simulink library "EngineModelsLibrary"  (R2014b)
settings: Solver=ode45  StartTime=0.0  StopTime=10.0  RelTol=1e-3
values from neighbouring files (symbols this model uses):
  k = 0.2    [ES_Run.m]    (also in ES_Run_v2.m = 10)
undefined symbols (not defined in the file or in its folder): b, COBRA_Compressor, cp, CPT_COBRA_LIB, D, etalim, gam, Newton, Pa, PARAM, Pl, pref, Ps, R, Raphson, rlim, T_0, Tref, Wclim
undefined symbols (not defined in the file): cr, e, etagain, fit_pars, kL, kS, par
(part 3 of 3)

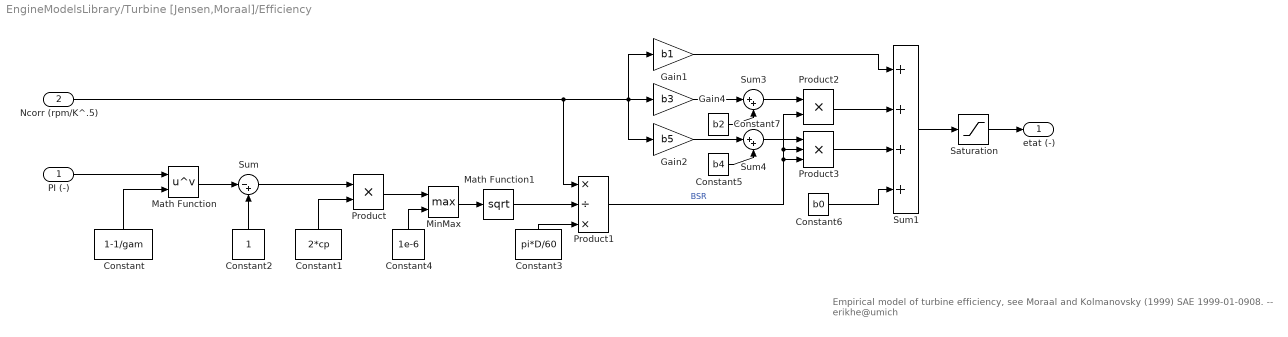
== system EngineModelsLibrary/Turbine [Jensen,Moraal]/Efficiency ==
  note: Empirical model of turbine efficiency, see Moraal and Kolmanovsky (1999) SAE 1999-01-0908.
      |  -- erikhe@umich
  PI (-) : Inport
  Ncorr (rpm/K^.5) : Inport  Port=2
  Constant : Constant  Value=1-1/gam
  Constant1 : Constant  Value=2*cp
  Constant2 : Constant
  Constant3 : Constant  Value=pi*D/60
  Constant4 : Constant  Value=1e-6
  Constant5 : Constant  Value=b4
  Constant6 : Constant  Value=b0
  Constant7 : Constant  Value=b2
  Gain1 : Gain  Gain=b1
  Gain2 : Gain  Gain=b5
  Gain4 : Gain  Gain=b3
  Math Function : Math  Operator=pow  SaturateOnIntegerOverflow=on
  Math Function1 : Math  Operator=sqrt  SaturateOnIntegerOverflow=on
  MinMax : MinMax  Function=max  Inputs=2
  Product : Product  RndMeth=Zero
  Product1 : Product  Inputs=*/*  RndMeth=Zero
  Product2 : Product  RndMeth=Zero
  Product3 : Product  Inputs=3  RndMeth=Zero
  Saturation : Saturate  UpperLimit=etamax  LowerLimit=etamin
  Sum : Sum  Inputs=|-+
  Sum1 : Sum  Inputs=4
  Sum3 : Sum  Inputs=|++
  Sum4 : Sum  Inputs=|++
  etat (-) : Outport
  wires:
  Product1/1 -> Product3/3, Product3/2, Product2/2  "BSR"
  Constant6/1 -> Sum1/4
  Product2/1 -> Sum1/2
  Product3/1 -> Sum1/3
  Sum4/1 -> Product3/1
  Sum3/1 -> Product2/1
  Gain1/1 -> Sum1/1
  Constant5/1 -> Sum4/2
  Constant7/1 -> Sum3/2
  Gain2/1 -> Sum4/1
  Gain4/1 -> Sum3/1
  Saturation/1 -> etat (-)/1
  Sum1/1 -> Saturation/1
  Ncorr (rpm/K^.5)/1 -> Gain1/1, Gain2/1, Gain4/1, Product1/1
  Constant3/1 -> Product1/3
  Constant4/1 -> MinMax/2
  Product/1 -> MinMax/1
  MinMax/1 -> Math Function1/1
  Math Function1/1 -> Product1/2
  Constant1/1 -> Product/2
  Constant2/1 -> Sum/2
  Math Function/1 -> Sum/1
  PI (-)/1 -> Math Function/1
  Constant/1 -> Math Function/2
  Sum/1 -> Product/1

== system EngineModelsLibrary/Turbine [Jensen,Moraal]/Mass flow ==
  note: Turbine mass flow as compressible flow through an orifice with variable effective area, see Jensen et al. SAE910070.
      | -- erikhe@umich
  pin (Pa) : Inport
  Tin (K) : Inport  Port=2
  PI (-) : Inport  Port=3
  Ncorr (rpm/K^.5) : Inport  Port=4
  Compressible flow : Subsystem
  Constant3 : Constant  Value=k22
  Constant7 : Constant  Value=k12
  Corrected flow inv : Subsystem
  Gain2 : Gain  Gain=k21
  Gain4 : Gain  Gain=k11
  Product1 : Product  Inputs=/*  RndMeth=Zero
  Saturation : Saturate  UpperLimit=Wtcmax  LowerLimit=Wtcmin
  Sum1 : Sum  Inputs=|++
  Sum3 : Sum  Inputs=|++
  Sum4 : Sum  Inputs=|++
  Wt (kg/s) : Outport
  wires:
  Compressible flow/1(mflow) -> Saturation/1
  Tin (K)/1 -> Corrected flow inv/1(Tin (K))
  Sum1/1 -> Compressible flow/2(Aeff)
  Product1/1 -> Sum1/1
  Sum4/1 -> Sum1/2  "kt2"
  Sum3/1 -> Product1/2  "kt1"
  Ncorr (rpm/K^.5)/1 -> Gain4/1, Gain2/1
  Constant3/1 -> Sum4/2
  Constant7/1 -> Sum3/2
  Gain2/1 -> Sum4/1
  Gain4/1 -> Sum3/1
  PI (-)/1 -> Product1/1, Compressible flow/1(PI (-))
  pin (Pa)/1 -> Corrected flow inv/2(pin (Pa))
  Corrected flow inv/1(Wt (kg/s)) -> Wt (kg/s)/1
  Saturation/1 -> Corrected flow inv/3(Wt corr (kg/s K^.5/Pa))

== system EngineModelsLibrary/Turbine [Jensen,Moraal]/Power ==
  W (kg/s) : Inport
  Tin (K) : Inport  Port=2
  Tout (K) : Inport  Port=3
  Constant : Constant  Value=cp
  Product : Product  Inputs=3  RndMeth=Zero
  Sum : Sum  Inputs=|+-
  P (W) : Outport
  wires:
  Tout (K)/1 -> Sum/2
  Tin (K)/1 -> Sum/1
  Constant/1 -> Product/3
  W (kg/s)/1 -> Product/1
  Sum/1 -> Product/2
  Product/1 -> P (W)/1

== system EngineModelsLibrary/Turbine [Jensen,Moraal]/Pressure ratio w saturation ==
  pin (Pa) : Inport
  pout (Pa) : Inport  Port=2
  Constant : Constant
  Divide : Product  Inputs=*/
  MinMax : MinMax  Inputs=2
  PI (-) : Outport
  wires:
  pout (Pa)/1 -> Divide/1
  pin (Pa)/1 -> Divide/2
  Divide/1 -> MinMax/1
  Constant/1 -> MinMax/2
  MinMax/1 -> PI (-)/1

== system EngineModelsLibrary/Turbine [Jensen,Moraal]/Temperature ==
  note: Temperature solved from the definition of efficiency. -- erikhe@umich
  PI (-) : Inport
  Tin (K) : Inport  Port=2
  etat (-) : Inport  Port=3
  Constant1 : Constant  Value=1-1/gam
  Constant2 : Constant
  Divide : Product  Inputs=**
  Divide1 : Product  Inputs=**
  Math Function : Math  Operator=pow  SaturateOnIntegerOverflow=on
  Sum : Sum  Inputs=+-|
  Sum1 : Sum  Inputs=+-|
  Tout (K) : Outport
  wires:
  PI (-)/1 -> Math Function/1
  Constant1/1 -> Math Function/2
  Sum/1 -> Divide/1
  etat (-)/1 -> Divide/2
  Sum1/1 -> Divide1/2
  Tin (K)/1 -> Divide1/1
  Divide1/1 -> Tout (K)/1
  Math Function/1 -> Sum/2
  Constant2/1 -> Sum1/1, Sum/1
  Divide/1 -> Sum1/2

== system EngineModelsLibrary/Turbine and wastegate/Turbine [Jensen,Moraal] ==
  pin (Pa) : Inport
  Tin (K) : Inport  Port=2
  w (rad/s) : Inport  Port=3
  pout (Pa) : Inport  Port=4
  Corrected speed : Subsystem
  Efficiency : Subsystem
  Gain : Gain  Gain=60
  Mass flow : Subsystem
  Power : Subsystem
  Pressure ratio w saturation : Subsystem
  Temperature : Subsystem
  Pt (W) : Outport
  etat (-) : Outport  Port=2
  Tt (K) : Outport  Port=3
  Wt (kg/s) : Outport  Port=4
  wires:
  Gain/1 -> Efficiency/2(Ncorr (rpm/K^.5)), Mass flow/4(Ncorr (rpm/K^.5))
  Power/1(P (W)) -> Pt (W)/1
  Efficiency/1(etat (-)) -> Temperature/3(etat (-)), etat (-)/1
  Temperature/1(Tout (K)) -> Power/3(Tout (K)), Tt (K)/1
  Mass flow/1(Wt (kg/s)) -> Power/1(W (kg/s)), Wt (kg/s)/1
  Corrected speed/1(Nc corr (rps/K^.5)) -> Gain/1
  Pressure ratio w saturation/1(PI (-)) -> Mass flow/3(PI (-)), Efficiency/1(PI (-)), Temperature/1(PI (-))
  pout (Pa)/1 -> Pressure ratio w saturation/2(pout (Pa))
  pin (Pa)/1 -> Pressure ratio w saturation/1(pin (Pa)), Mass flow/1(pin (Pa))
  Tin (K)/1 -> Temperature/2(Tin (K)), Power/2(Tin (K)), Mass flow/2(Tin (K)), Corrected speed/1(Tin (K))
  w (rad/s)/1 -> Corrected speed/2(w (rad/s))

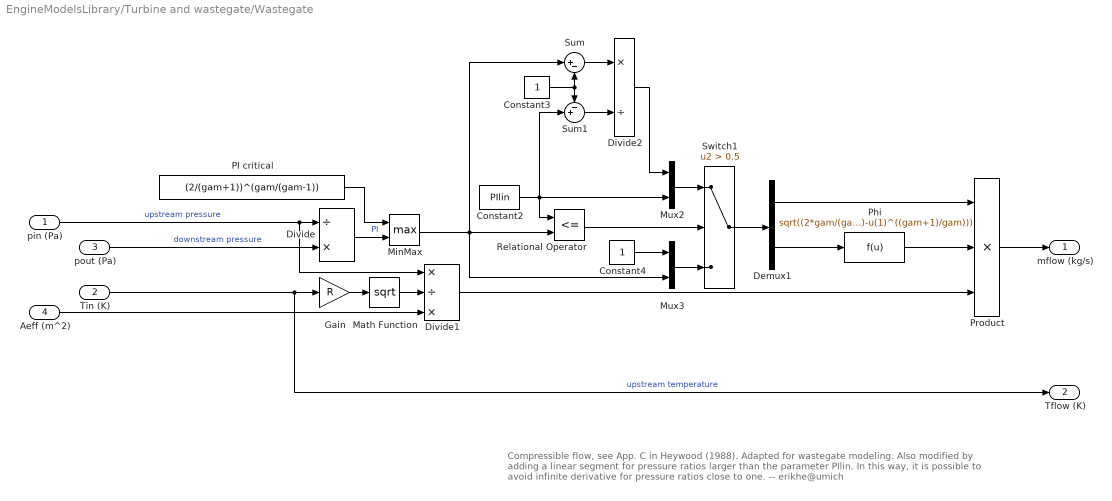
== system EngineModelsLibrary/Turbine and wastegate/Wastegate ==
  note: Compressible flow, see App. C in Heywood (1988). Adapted for wastegate modeling. Also modified by adding a linear segment for pressure ratios larger than
      | the parameter PIlin. In this way, it is possible to avoid infinite derivative for pressure ratios close to one. -- erikhe@umich
  pin (Pa) : Inport
  Tin (K) : Inport  Port=2
  pout (Pa) : Inport  Port=3
  Aeff (m^2) : Inport  Port=4
  Constant2 : Constant  Value=PIlin
  Constant3 : Constant
  Constant4 : Constant
  Demux1 : Demux  Outputs=2
  Divide : Product  Inputs=/*
  Divide1 : Product  Inputs=*/*
  Divide2 : Product  Inputs=*/
  Gain : Gain  Gain=R
  Math Function : Math  Operator=sqrt  SaturateOnIntegerOverflow=on
  MinMax : MinMax  Function=max  Inputs=2
  Mux2 : Mux  Inputs=2
  Mux3 : Mux  Inputs=2
  PI critical : Constant  Value=(2/(gam+1))^(gam/(gam-1))
  Phi : Fcn  Expr=sqrt((2*gam/(gam-1))*(u(1)^(2/gam)-u(1)^((gam+1)/gam)))
  Product : Product  Inputs=3  RndMeth=Zero
  Relational Operator : RelationalOperator  Operator=<=  OutDataTypeStr=boolean
  Sum : Sum  Inputs=|+-
  Sum1 : Sum  Inputs=-+|
  Switch1 : Switch  Criteria=u2 > Threshold  Threshold=0.5
  mflow (kg/s) : Outport
  Tflow (K) : Outport  Port=2
  wires:
  Phi/1 -> Product/2
  Demux1/1 -> Product/1
  Demux1/2 -> Phi/1
  Switch1/1 -> Demux1/1
  Constant4/1 -> Mux3/1
  Mux3/1 -> Switch1/3
  Mux2/1 -> Switch1/1
  Divide2/1 -> Mux2/1
  Sum1/1 -> Divide2/2
  Sum/1 -> Divide2/1
  Constant3/1 -> Sum1/1, Sum/2
  Relational Operator/1 -> Switch1/2
  Constant2/1 -> Sum1/2, Mux2/2, Relational Operator/1
  MinMax/1 -> Sum/1, Mux3/2, Relational Operator/2
  pin (Pa)/1 -> Divide/1, Divide1/1  "upstream pressure"
  pout (Pa)/1 -> Divide/2  "downstream pressure"
  Divide/1 -> MinMax/2  "PI"
  Tin (K)/1 -> Gain/1, Tflow (K)/1  "upstream temperature"
  PI critical/1 -> MinMax/1
  Gain/1 -> Math Function/1
  Aeff (m^2)/1 -> Divide1/3
  Math Function/1 -> Divide1/2
  Divide1/1 -> Product/3
  Product/1 -> mflow (kg/s)/1

== system EngineModelsLibrary/Wastegate Flow /Get Critical WG signal ==
  P_emr (Pa) : Inport
  P_ex (Pa) : Inport  Port=2
  Add : Sum  Inputs=+-+
  Add1 : Sum
  Constant : Constant  Value=Ps
  Constant1 : Constant  Value=k
  Constant2 : Constant  Value=Pa
  Constant3 : Constant  Value=Pl
  Divide : Product  Inputs=*/
  Divide1 : Product  Inputs=*/
  Gain : Gain  Gain=1e-3
  Gain1 : Gain  Gain=1e-3
  u_crit (-) : Outport
  wires:
  Gain1/1 -> Add/2
  Gain/1 -> Add/3
  Divide1/1 -> u_crit (-)/1
  Constant3/1 -> Divide1/2
  Add1/1 -> Divide1/1
  Constant2/1 -> Add1/2
  Divide/1 -> Add1/1
  Constant1/1 -> Divide/2
  Add/1 -> Divide/1
  Constant/1 -> Add/1
  P_ex (Pa)/1 -> Gain/1
  P_emr (Pa)/1 -> Gain1/1

== system EngineModelsLibrary/Wastegate Flow /Orifice flow ==
  Pi_wg (-) : Inport
  Add3 : Sum  Inputs=+-
  Math Function : Math  Operator=pow  SaturateOnIntegerOverflow=on
  Math Function1 : Math  Operator=pow  SaturateOnIntegerOverflow=on
  MinMax : MinMax  Function=max  Inputs=2
  Product : Product  RndMeth=Zero
  Sqrt : Sqrt  SaturateOnIntegerOverflow=on
  choked flow pressure ratio : Constant  Value=(2/(gam+1))^(gam/(gam-1))
  "exp 1 " : Constant  Value=2/gam
  exp 2 : Constant  Value=(gam+1)/gam
  "multiplier " : Constant  Value=2*gam/(gam-1)
  Psi (-) : Outport
  wires:
  choked flow pressure ratio/1 -> MinMax/2
  Pi_wg (-)/1 -> MinMax/1
  Sqrt/1 -> Psi (-)/1
  Product/1 -> Sqrt/1
  Add3/1 -> Product/2
  "multiplier "/1 -> Product/1
  Math Function1/1 -> Add3/2
  Math Function/1 -> Add3/1
  exp 2/1 -> Math Function1/2
  MinMax/1 -> Math Function/1, Math Function1/1
  "exp 1 "/1 -> Math Function/2

== system EngineModelsLibrary/Wastegate Flow /Wastegate Area  ==
  u-u_crit (%) : Inport
  Pressure ratio (-) : Inport  Port=2
  Add : Sum
  Add1 : Sum
  Add2 : Sum  Inputs=+-
  Constant : Constant  Value=c(1)
  Constant1 : Constant  Value=c(2)
  Constant2 : Constant  Value=c(3)
  Constant3 : Constant  Value=c(4)
  Constant4 : Constant
  Constant5 : Constant  Value=2
  Constant6 : Constant
  Divide : Product  Inputs=*/
  Divide1 : Product  Inputs=*/
  Gain : Gain  Gain=-1
  Math Function : Math  SaturateOnIntegerOverflow=on
  Product : Product  RndMeth=Zero
  Product1 : Product  Inputs=3  RndMeth=Zero
  A (m^2) : Outport
  wires:
  Product1/1 -> A (m^2)/1
  Add2/1 -> Product1/2
  Constant6/1 -> Add2/2
  Divide1/1 -> Add2/1
  Constant5/1 -> Divide1/1
  Add1/1 -> Divide1/2
  Constant4/1 -> Add1/1
  Math Function/1 -> Add1/2
  Gain/1 -> Math Function/1
  Divide/1 -> Gain/1
  u-u_crit (%)/1 -> Divide/1
  Constant1/1 -> Divide/2
  Constant/1 -> Product1/1
  Add/1 -> Product1/3
  Constant3/1 -> Add/2
  Product/1 -> Add/1
  Constant2/1 -> Product/2
  Pressure ratio (-)/1 -> Product/1

== system EngineModelsLibrary/Compressor [Eriksson]/Mass flow/Density ==
  p (Pa) : Inport
  T (K) : Inport  Port=2
  Constant1 : Constant  Value=R
  Product : Product  Inputs=*//  RndMeth=Zero
  rho (kg/m^3) : Outport
  wires:
  p (Pa)/1 -> Product/1
  T (K)/1 -> Product/2
  Constant1/1 -> Product/3
  Product/1 -> rho (kg/m^3)/1

== system EngineModelsLibrary/Compressor [Jensen simplified]/Mass flow/Density ==
  p (Pa) : Inport
  T (K) : Inport  Port=2
  Constant1 : Constant  Value=R
  Product : Product  Inputs=*//  RndMeth=Zero
  rho (kg/m^3) : Outport
  wires:
  Product/1 -> rho (kg/m^3)/1
  Constant1/1 -> Product/3
  T (K)/1 -> Product/2
  p (Pa)/1 -> Product/1

== system EngineModelsLibrary/Large scroll turbine/Mass flow/Corrected flow inv ==
  note: Inversion of mass flow corrected based on inlet conditions.
      | -- erikhe@umich
  Pin (bar) : Inport
  Tin (K) : Inport  Port=2
  Wt corr (kg/s K^.5/bar) : Inport  Port=3
  Divide3 : Product  Inputs=/**
  Math Function : Math  Operator=sqrt  SaturateOnIntegerOverflow=on
  Wt (kg/s) : Outport
  wires:
  Divide3/1 -> Wt (kg/s)/1
  Wt corr (kg/s K^.5/bar)/1 -> Divide3/2
  Pin (bar)/1 -> Divide3/3
  Math Function/1 -> Divide3/1
  Tin (K)/1 -> Math Function/1

== system EngineModelsLibrary/Small scroll turbine/Mass flow/Corrected flow inv ==
  note: Inversion of mass flow corrected based on inlet conditions.
      | -- erikhe@umich
  Pin (bar) : Inport
  Tin (K) : Inport  Port=2
  Wt corr (kg/s K^.5/bar) : Inport  Port=3
  Divide3 : Product  Inputs=/**
  Math Function : Math  Operator=sqrt  SaturateOnIntegerOverflow=on
  Wt (kg/s) : Outport
  wires:
  Tin (K)/1 -> Math Function/1
  Math Function/1 -> Divide3/1
  Pin (bar)/1 -> Divide3/3
  Wt corr (kg/s K^.5/bar)/1 -> Divide3/2
  Divide3/1 -> Wt (kg/s)/1

== system EngineModelsLibrary/Turbine [Eriksson]/Mass flow/Corrected flow inv ==
  note: Mass flow corrected based on inlet conditions and reference state.
      | -- erikhe@umich
  pin (Pa) : Inport
  Tin (K) : Inport  Port=2
  Wcorr (kg/s) : Inport  Port=3
  Constant : Constant  Value=Tref
  Constant2 : Constant  Value=pref
  Divide : Product  Inputs=*/
  Divide2 : Product  Inputs=*/
  Divide3 : Product  Inputs=/**
  Math Function : Math  Operator=sqrt  SaturateOnIntegerOverflow=on
  W (kg/s) : Outport
  wires:
  Divide/1 -> Math Function/1
  Constant/1 -> Divide/2
  Tin (K)/1 -> Divide/1
  Math Function/1 -> Divide3/1
  Constant2/1 -> Divide2/2
  pin (Pa)/1 -> Divide2/1
  Divide2/1 -> Divide3/3
  Wcorr (kg/s)/1 -> Divide3/2
  Divide3/1 -> W (kg/s)/1

== system EngineModelsLibrary/Turbine [Jensen,Moraal]/Mass flow/Compressible flow ==
  note: Isentropic compressible flow, see App. C in Heywood (1988). Adapted for turbine mass flow modeling. Also modified by adding a linear segment for pressure ratios larger than
      | the parameter PIlin. In this way, it is possible to avoid infinite derivative for pressure ratios close to one. -- erikhe@umich
  PI (-) : Inport
  Aeff : Inport  Port=2
  Constant2 : Constant  Value=PIlin
  Constant3 : Constant
  Constant4 : Constant
  Demux1 : Demux  Outputs=2
  Divide2 : Product  Inputs=*/
  MinMax : MinMax  Function=max  Inputs=2
  Mux2 : Mux  Inputs=2
  Mux3 : Mux  Inputs=2
  PI critical : Constant  Value=(2/(gam+1))^(gam/(gam-1))
  Phi : Fcn  Expr=sqrt((2*gam/(gam-1))*(u(1)^(2/gam)-u(1)^((gam+1)/gam)))
  Product : Product  Inputs=3  RndMeth=Zero
  Relational Operator : RelationalOperator  Operator=<=  OutDataTypeStr=boolean
  Sum : Sum  Inputs=|+-
  Sum1 : Sum  Inputs=-+|
  Switch1 : Switch  Criteria=u2 > Threshold  Threshold=0.5
  mflow : Outport
  wires:
  Phi/1 -> Product/2
  Demux1/1 -> Product/1
  Demux1/2 -> Phi/1
  Switch1/1 -> Demux1/1
  Constant4/1 -> Mux3/1
  Mux3/1 -> Switch1/3
  Mux2/1 -> Switch1/1
  Divide2/1 -> Mux2/1
  Sum1/1 -> Divide2/2
  Sum/1 -> Divide2/1
  Constant3/1 -> Sum1/1, Sum/2
  Relational Operator/1 -> Switch1/2
  Constant2/1 -> Sum1/2, Mux2/2, Relational Operator/1
  MinMax/1 -> Sum/1, Mux3/2, Relational Operator/2
  PI (-)/1 -> MinMax/2
  PI critical/1 -> MinMax/1
  Aeff/1 -> Product/3
  Product/1 -> mflow/1

== system EngineModelsLibrary/Turbine [Jensen,Moraal]/Mass flow/Corrected flow inv ==
  note: Inversion of mass flow corrected based on inlet conditions.
      | -- erikhe@umich
  Tin (K) : Inport
  pin (Pa) : Inport  Port=2
  Wt corr (kg/s K^.5/Pa) : Inport  Port=3
  Divide3 : Product  Inputs=/**
  Math Function : Math  Operator=sqrt  SaturateOnIntegerOverflow=on
  Wt (kg/s) : Outport
  wires:
  Divide3/1 -> Wt (kg/s)/1
  Wt corr (kg/s K^.5/Pa)/1 -> Divide3/2
  pin (Pa)/1 -> Divide3/3
  Math Function/1 -> Divide3/1
  Tin (K)/1 -> Math Function/1

== system EngineModelsLibrary/Turbine and wastegate/Turbine [Jensen,Moraal]/Corrected speed ==
  note: Speed corrected based on inlet conditions.
      | -- erikhe@umich
  Tin (K) : Inport
  w (rad/s) : Inport  Port=2
  Divide1 : Product  Inputs=*/
  Gain : Gain  Gain=1/(2*pi)
  Math Function : Math  Operator=sqrt  SaturateOnIntegerOverflow=on
  Nc corr (rps/K^.5) : Outport
  wires:
  Gain/1 -> Divide1/1
  Divide1/1 -> Nc corr (rps/K^.5)/1
  Math Function/1 -> Divide1/2
  w (rad/s)/1 -> Gain/1
  Tin (K)/1 -> Math Function/1

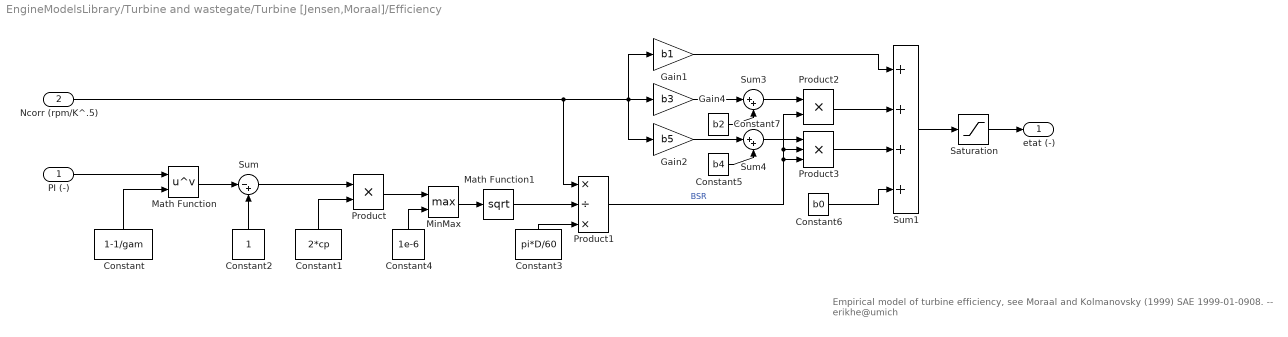
== system EngineModelsLibrary/Turbine and wastegate/Turbine [Jensen,Moraal]/Efficiency ==
  note: Empirical model of turbine efficiency, see Moraal and Kolmanovsky (1999) SAE 1999-01-0908.
      |  -- erikhe@umich
  PI (-) : Inport
  Ncorr (rpm/K^.5) : Inport  Port=2
  Constant : Constant  Value=1-1/gam
  Constant1 : Constant  Value=2*cp
  Constant2 : Constant
  Constant3 : Constant  Value=pi*D/60
  Constant4 : Constant  Value=1e-6
  Constant5 : Constant  Value=b4
  Constant6 : Constant  Value=b0
  Constant7 : Constant  Value=b2
  Gain1 : Gain  Gain=b1
  Gain2 : Gain  Gain=b5
  Gain4 : Gain  Gain=b3
  Math Function : Math  Operator=pow  SaturateOnIntegerOverflow=on
  Math Function1 : Math  Operator=sqrt  SaturateOnIntegerOverflow=on
  MinMax : MinMax  Function=max  Inputs=2
  Product : Product  RndMeth=Zero
  Product1 : Product  Inputs=*/*  RndMeth=Zero
  Product2 : Product  RndMeth=Zero
  Product3 : Product  Inputs=3  RndMeth=Zero
  Saturation : Saturate  UpperLimit=etamax  LowerLimit=etamin
  Sum : Sum  Inputs=|-+
  Sum1 : Sum  Inputs=4
  Sum3 : Sum  Inputs=|++
  Sum4 : Sum  Inputs=|++
  etat (-) : Outport
  wires:
  Sum/1 -> Product/1
  Constant/1 -> Math Function/2
  PI (-)/1 -> Math Function/1
  Math Function/1 -> Sum/1
  Constant2/1 -> Sum/2
  Constant1/1 -> Product/2
  Math Function1/1 -> Product1/2
  MinMax/1 -> Math Function1/1
  Product/1 -> MinMax/1
  Constant4/1 -> MinMax/2
  Constant3/1 -> Product1/3
  Ncorr (rpm/K^.5)/1 -> Product1/1, Gain4/1, Gain2/1, Gain1/1
  Sum1/1 -> Saturation/1
  Saturation/1 -> etat (-)/1
  Gain4/1 -> Sum3/1
  Gain2/1 -> Sum4/1
  Constant7/1 -> Sum3/2
  Constant5/1 -> Sum4/2
  Gain1/1 -> Sum1/1
  Sum3/1 -> Product2/1
  Sum4/1 -> Product3/1
  Product3/1 -> Sum1/3
  Product2/1 -> Sum1/2
  Constant6/1 -> Sum1/4
  Product1/1 -> Product2/2, Product3/2, Product3/3  "BSR"

== system EngineModelsLibrary/Turbine and wastegate/Turbine [Jensen,Moraal]/Mass flow ==
  note: Turbine mass flow as compressible flow through an orifice with variable effective area, see Jensen et al. SAE910070.
      | -- erikhe@umich
  pin (Pa) : Inport
  Tin (K) : Inport  Port=2
  PI (-) : Inport  Port=3
  Ncorr (rpm/K^.5) : Inport  Port=4
  Compressible flow : Subsystem
  Constant3 : Constant  Value=k22
  Constant7 : Constant  Value=k12
  Corrected flow inv : Subsystem
  Gain2 : Gain  Gain=k21
  Gain4 : Gain  Gain=k11
  Product1 : Product  Inputs=/*  RndMeth=Zero
  Saturation : Saturate  UpperLimit=Wtcmax  LowerLimit=Wtcmin
  Sum1 : Sum  Inputs=|++
  Sum3 : Sum  Inputs=|++
  Sum4 : Sum  Inputs=|++
  Wt (kg/s) : Outport
  wires:
  Saturation/1 -> Corrected flow inv/3(Wt corr (kg/s K^.5/Pa))
  Corrected flow inv/1(Wt (kg/s)) -> Wt (kg/s)/1
  pin (Pa)/1 -> Corrected flow inv/2(pin (Pa))
  PI (-)/1 -> Compressible flow/1(PI (-)), Product1/1
  Gain4/1 -> Sum3/1
  Gain2/1 -> Sum4/1
  Constant7/1 -> Sum3/2
  Constant3/1 -> Sum4/2
  Ncorr (rpm/K^.5)/1 -> Gain2/1, Gain4/1
  Sum3/1 -> Product1/2  "kt1"
  Sum4/1 -> Sum1/2  "kt2"
  Product1/1 -> Sum1/1
  Sum1/1 -> Compressible flow/2(Aeff)
  Tin (K)/1 -> Corrected flow inv/1(Tin (K))
  Compressible flow/1(mflow) -> Saturation/1

== system EngineModelsLibrary/Turbine and wastegate/Turbine [Jensen,Moraal]/Power ==
  W (kg/s) : Inport
  Tin (K) : Inport  Port=2
  Tout (K) : Inport  Port=3
  Constant : Constant  Value=cp
  Product : Product  Inputs=3  RndMeth=Zero
  Sum : Sum  Inputs=|+-
  P (W) : Outport
  wires:
  Product/1 -> P (W)/1
  Sum/1 -> Product/2
  W (kg/s)/1 -> Product/1
  Constant/1 -> Product/3
  Tin (K)/1 -> Sum/1
  Tout (K)/1 -> Sum/2

== system EngineModelsLibrary/Turbine and wastegate/Turbine [Jensen,Moraal]/Pressure ratio w saturation ==
  pin (Pa) : Inport
  pout (Pa) : Inport  Port=2
  Constant : Constant
  Divide : Product  Inputs=*/
  MinMax : MinMax  Inputs=2
  PI (-) : Outport
  wires:
  MinMax/1 -> PI (-)/1
  Constant/1 -> MinMax/2
  Divide/1 -> MinMax/1
  pin (Pa)/1 -> Divide/2
  pout (Pa)/1 -> Divide/1

== system EngineModelsLibrary/Turbine and wastegate/Turbine [Jensen,Moraal]/Temperature ==
  note: Temperature solved from the definition of efficiency. -- erikhe@umich
  PI (-) : Inport
  Tin (K) : Inport  Port=2
  etat (-) : Inport  Port=3
  Constant1 : Constant  Value=1-1/gam
  Constant2 : Constant
  Divide : Product  Inputs=**
  Divide1 : Product  Inputs=**
  Math Function : Math  Operator=pow  SaturateOnIntegerOverflow=on
  Sum : Sum  Inputs=+-|
  Sum1 : Sum  Inputs=+-|
  Tout (K) : Outport
  wires:
  Divide/1 -> Sum1/2
  Constant2/1 -> Sum/1, Sum1/1
  Math Function/1 -> Sum/2
  Divide1/1 -> Tout (K)/1
  Tin (K)/1 -> Divide1/1
  Sum1/1 -> Divide1/2
  etat (-)/1 -> Divide/2
  Sum/1 -> Divide/1
  Constant1/1 -> Math Function/2
  PI (-)/1 -> Math Function/1

== system EngineModelsLibrary/Turbine and wastegate/Turbine [Jensen,Moraal]/Mass flow/Compressible flow ==
  note: Isentropic compressible flow, see App. C in Heywood (1988). Adapted for turbine mass flow modeling. Also modified by adding a linear segment for pressure ratios larger than
      | the parameter PIlin. In this way, it is possible to avoid infinite derivative for pressure ratios close to one. -- erikhe@umich
  PI (-) : Inport
  Aeff : Inport  Port=2
  Constant2 : Constant  Value=PIlin
  Constant3 : Constant
  Constant4 : Constant
  Demux1 : Demux  Outputs=2
  Divide2 : Product  Inputs=*/
  MinMax : MinMax  Function=max  Inputs=2
  Mux2 : Mux  Inputs=2
  Mux3 : Mux  Inputs=2
  PI critical : Constant  Value=(2/(gam+1))^(gam/(gam-1))
  Phi : Fcn  Expr=sqrt((2*gam/(gam-1))*(u(1)^(2/gam)-u(1)^((gam+1)/gam)))
  Product : Product  Inputs=3  RndMeth=Zero
  Relational Operator : RelationalOperator  Operator=<=  OutDataTypeStr=boolean
  Sum : Sum  Inputs=|+-
  Sum1 : Sum  Inputs=-+|
  Switch1 : Switch  Criteria=u2 > Threshold  Threshold=0.5
  mflow : Outport
  wires:
  Product/1 -> mflow/1
  Aeff/1 -> Product/3
  PI critical/1 -> MinMax/1
  PI (-)/1 -> MinMax/2
  MinMax/1 -> Relational Operator/2, Mux3/2, Sum/1
  Constant2/1 -> Relational Operator/1, Mux2/2, Sum1/2
  Relational Operator/1 -> Switch1/2
  Constant3/1 -> Sum/2, Sum1/1
  Sum/1 -> Divide2/1
  Sum1/1 -> Divide2/2
  Divide2/1 -> Mux2/1
  Mux2/1 -> Switch1/1
  Mux3/1 -> Switch1/3
  Constant4/1 -> Mux3/1
  Switch1/1 -> Demux1/1
  Demux1/2 -> Phi/1
  Demux1/1 -> Product/1
  Phi/1 -> Product/2

== system EngineModelsLibrary/Turbine and wastegate/Turbine [Jensen,Moraal]/Mass flow/Corrected flow inv ==
  note: Inversion of mass flow corrected based on inlet conditions.
      | -- erikhe@umich
  Tin (K) : Inport
  pin (Pa) : Inport  Port=2
  Wt corr (kg/s K^.5/Pa) : Inport  Port=3
  Divide3 : Product  Inputs=/**
  Math Function : Math  Operator=sqrt  SaturateOnIntegerOverflow=on
  Wt (kg/s) : Outport
  wires:
  Tin (K)/1 -> Math Function/1
  Math Function/1 -> Divide3/1
  pin (Pa)/1 -> Divide3/3
  Wt corr (kg/s K^.5/Pa)/1 -> Divide3/2
  Divide3/1 -> Wt (kg/s)/1
